simulink model "model_linear_2019"  (R2019a)
settings: Solver=VariableStepAuto  StartTime=0.0  StopTime=20  RelTol=1e-3
values from neighbouring files (symbols this model uses):
  beta_r = deg2rad(beta)    [params.m]
  g = 9.81    [params.m]
  Jz = rl^2 * (1/3 * mbL + ml) + rp^2 * (1/3 * mbP + mp)    [inertia.m]
  mw = 0.0256 * 1.5    (= 0.0384)    [params.m]
  rw = 0.270    (= 0.27)    [params.m]
settings Model: Creator=Kamil  LastModifiedBy=Kamil
settings DebuggingCC: UnconnectedInputMsg=none  UnconnectedOutputMsg=none  UnconnectedLineMsg=none  SFMachineParentedDataDiag=error

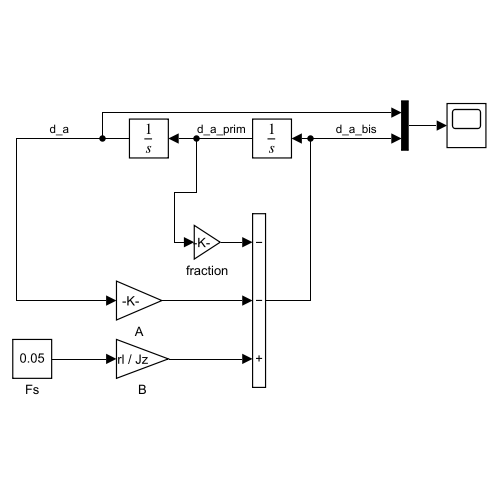
[thumbnail: Simulink's stored preview of the top-level diagram]
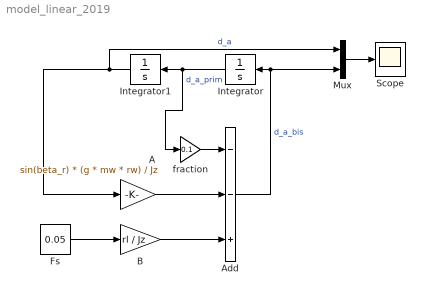
== system model_linear_2019 ==
  A : Gain  Gain=sin(beta_r) * (g * mw * rw) / Jz
  Add : Sum  Inputs=--+
  B : Gain  Gain=rl / Jz
  Fs : Constant  Value=0.05  VectorParams1D=off
  Integrator : Integrator
  Integrator1 : Integrator
  Mux : Mux  Inputs=2
  Scope : Scope
  fraction : Gain  Gain=0.1
  wires:
  Mux/1 -> Scope/1
  Integrator/1 -> fraction/1, Integrator1/1  "d_a_prim"
  A/1 -> Add/2
  B/1 -> Add/3
  Fs/1 -> B/1
  Add/1 -> Mux/2, Integrator/1  "d_a_bis"
  Integrator1/1 -> Mux/1, A/1  "d_a"
  fraction/1 -> Add/1
